simulink library "rappid_564xl_ec_toolbox"  (R2016b)
settings: Solver=FixedStepDiscrete  StartTime=0.0  StopTime=10.0  RelTol=1e-3  EnableMultiTasking=on
undefined symbols (not defined in the file or in its folder): CTU_unit, mem_AddrLW, mem_AddrUP, rappid_564xl_adc_input_support_rev2, rappid_564xl_can_support_rev2, read_mem_AddrLW, read_mem_AddrUP
(part 3 of 6)

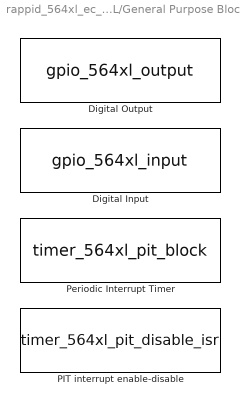
== system rappid_564xl_ec_toolbox/MPC564xL/General Purpose Blocks ==
  Digital Input : S-Function  FunctionName=gpio_564xl_input  Parameters=uint16(pcrNum)  SFunctionDeploymentMode=off  EnableBusSupport=off  mask(GPIO_564xL_Input){gpio_outputs=None, pinNum=None Selected, pcrNum=}
      mask prompts: gpio_outputs "Output Pin (GPI [0-144])"; pinNum "Pin Number"; pcrNum "PCR Number"
      mask help:
      | Select a General Purpose Input Pin as a Source.
      | Output Legend (PCR : Port Name : [ Pin# 144pkg ] : [ Pin# 257pkg ])
      mask init:
      | gpioInfoOut = rappid_564xl_get_gpio_info(gcb);
      | set_param(gcb,'pinNum',gpioInfoOut.pinNum);
      | set_param(gcb,'pcrNum',gpioInfoOut.pcrNum);
      | st=['Pin: ', gpioInfoOut.pinNum,' ',gpioInfoOut.portName,' '];
      mask Help: web([rappid_block_help,filesep,'gpio_input.htm']);
      mask TypeOptions gpio_outputs: 0   : PA0  : [ 73 ] : [ T14 ] | 1   : PA1  : [ 74 ] : [ R14 ] | 2   : PA2  : [ 84 ] : [ N16 ] | 3   : PA3  : [ 92 ] : [ K17 ] | 4   : PA4  : [ 108 ] : [ C16 ] | 5   : PA5  : [ 14 ] : [ H4 ] | 6   : PA6  : [ 2 ] : [ G4 ] | 7   : PA7  : [ 10 ] : [ F3 ] | 8   : PA8  : [ 12 ] : [ F4 ] | 9   : PA9  : [ 134 ] : [ B6 ] | 10  : PA10  : [ 118 ] : [ A13 ] | 11  : PA11 : [ 120 ] : [ D11 ] | 12  : PA12 : [ 122 ] : [ A10 ] | 13  : PA13 : [ 136 ] : [ C6 ] | 14  : PA14 : [ 143 ] : [ B4 ] | 15  : PA15 : [ 144 ] : [ D3 ] | 16  : PB0  : [ 109 ] : [ B15 ] | 17  : PB1  : [ 110 ] : [ C14 ] | 18  : PB2  : [ 114 ] : [ A14 ] | 19  : PB3  : [ 116 ] : [ B13 ] | 20  : PB4  : [ 89 ] : [ L17 ] | 21  : PB5  : [ 86 ] : [ M15 ] | 22  : PB6  : [ 138 ] : [ B3 ] | 23  : PB7  : [ 43 ] : [ R5 ] | 24  : PB8  : [ 47 ] : [ P7 ] | 25  : PB9  : [ 52 ] : [ U7 ] | 26  : PB10 : [ 53 ] : [ R8 ] | 27  : PB11 : [ 54 ] : [ T8 ] | 28  : PB12 : [ 55 ] : [ U8 ] | 29  : PB13 : [ 60 ] : [ R10 ] | 30  : PB14 : [ 64 ] : [ P11 ] | 31  : PB15 : [ 62 ] : [ R11 ] | 32  : PC0  : [ 66 ] : [ R12 ] | 33  : PC1  : [ 41 ] : [ T4 ] | 34  : PC2  : [ 45 ] : [ U5 ] | 36  : PC4  : [ 11 ] : [ H3 ] | 37  : PC5  : [ 13 ] : [ G3 ] | 38  : PC6  : [ 142 ] : [ D4 ] | 39  : PC7  : [ 15 ] : [ K4 ] | 42  : PC10 : [ 111 ] : [ A15 ] | 43  : PC11 : [ 80 ] : [ M14 ] | 44  : PC12 : [ 82 ] : [ N15 ] | 45  : PC13 : [ 101 ] : [ F15 ] | 46  : PC14 : [ 103 ] : [ E15 ] | 47  : PC15 : [ 124 ] : [ A8 ] | 48  : PD0  : [ 125 ] : [ B8 ] | 49  : PD1  : [ 3 ] : [ E3 ] | 50  : PD2  : [ 140 ] : [ C5 ] | 51  : PD3  : [ 128 ] : [ A7 ] | 52  : PD4  : [ 129 ] : [ B7 ] | 53  : PD5  : [ 33 ] : [ N3 ] | 54  : PD6  : [ 34 ] : [ P3 ] | 55  : PD7  : [ 37 ] : [ R4 ] | 56  : PD8  : [ 32 ] : [ M3 ] | 57  : PD9  : [ 26 ] : [ L3 ] | 58  : PD10 : [ 76 ] : [ T15 ] | 59  : PD11 : [ 78 ] : [ R16 ] | 60  : PD12 : [ 99 ] : [ G14 ] | 62  : PD14 : [ 105 ] : [ D16 ] | 64  : PE0  : [ 68 ] : [ T13 ] | 66  : PE2  : [ 49 ] : [ U6 ] | 68  : PE4  : [ 42 ] : [ U4 ] | 69  : PE5  : [ 44 ] : [ T5 ] | 70  : PE6  : [ 46 ] : [ R6 ] | 71  : PE7  : [ 48 ] : [ T6 ] | 73  : PE9  : [ 61 ] : [ T10 ] | 74  : PE10 : [ 63 ] : [ T11 ] | 75  : PE11 : [ 65 ] : [ U11 ] | 76  : PE12 : [ 67 ] : [ T12 ] | 77  : PE13 : [ 117 ] : [ D12 ] | 78  : PE14 : [ 119 ] : [ B12 ] | 79  : PE15 : [ 121 ] : [ B11 ] | 80  : PF0  : [ 133 ] : [ D7 ] | 83  : PF3  : [ 139 ] : [ B5 ] | 84  : PF4  : [ 4 ] : [ D2 ] | 85  : PF5  : [ 5 ] : [ D1 ] | 86  : PF6  : [ 8 ] : [ E2 ] | 87  : PF7  : [ 19 ] : [ J1 ] | 88  : PF8  : [ 20 ] : [ K2 ] | 89  : PF9  : [ 23 ] : [ K1 ] | 90  : PF10 : [ 24 ] : [ L1 ] | 91  : PF11 : [ 25 ] : [ L2 ] | 92  : PF12 : [ 106 ] : [ C17 ] | 93  : PF13 : [ 112 ] : [ B14 ] | 94  : PF14 : [ 115 ] : [ C13 ] | 95  : PF15 : [ 113 ] : [ D13 ] | 98  : PG2  : [ 102 ] : [ E16 ] | 99  : PG3  : [ 104 ] : [ D17 ] | 100 : PG4  : [ 100 ] : [ F17 ] | 101 : PG5  : [ 85 ] : [ N17 ] | 102 : PG6  : [ 98 ] : [ G17 ] | 103 : PG7  : [ 83 ] : [ P17 ] | 104 : PG8  : [ 81 ] : [ P16 ] | 105 : PG9  : [ 79 ] : [ R17 ] | 106 : PG10 : [ 77 ] : [ P15 ] | 107 : PG11 : [ 75 ] : [ U15 ] | 108 : PG12 : [ --- ] : [ F2 ] | 109 : PG13 : [ --- ] : [ H1 ] | 110 : PG14 : [ --- ] : [ A6 ] | 111 : PG15 : [ --- ] : [ J2 ] | 112 : PH0  : [ --- ] : [ A5 ] | 113 : PH1  : [ --- ] : [ F1 ] | 114 : PH2  : [ --- ] : [ A4 ] | 115 : PH3  : [ --- ] : [ G1 ] | 116 : PH4  : [ --- ] : [ L16 ] | 117 : PH5  : [ --- ] : [ M17 ] | 118 : PH6  : [ --- ] : [ H17 ] | 119 : PH7  : [ --- ] : [ K16 ] | 120 : PH8  : [ --- ] : [ K15 ] | 121 : PH9  : [ --- ] : [ G16 ] | 122 : PH10 : [ --- ] : [ A11 ] | 123 : PH11 : [ --- ] : [ C11 ] | 124 : PH12 : [ --- ] : [ B10 ] | 125 : PH13 : [ --- ] : [ G15 ] | 126 : PH14 : [ --- ] : [ A12 ] | 127 : PH15 : [ --- ] : [ J17 ] | 128 : PI0  : [ --- ] : [ C9 ] | 129 : PI1  : [ --- ] : [ C12 ] | 130 : PI2  : [ --- ] : [ F16 ] | 131 : PI3  : [ --- ] : [ E17 ] | 132 : PI4  : [ --- ] : [ K3 ] | None
      mask Display:
      | disp(st);
      | port_label('output',1,'input')
  "Digital Output " : S-Function  FunctionName=gpio_564xl_output  Parameters=uint16(pcrNum)  SFunctionDeploymentMode=off  EnableBusSupport=off  mask(GPIO_564xL_Output){gpio_outputs=None, pinNum=None Selected, pcrNum=}
      mask prompts: gpio_outputs "Output Pin (GPO [0-144])"; pinNum "Pin Number"; pcrNum "PCR Number"
      mask help:
      | Select a General Purpose Output Pin as a Sink.
      | Output Legend (PCR : Port Name : [ Pin# 144pkg ] : [ Pin# 257pkg ])
      mask init:
      | gpioInfoOut = rappid_564xl_get_gpio_info(gcb);
      | set_param(gcb,'pinNum',gpioInfoOut.pinNum);
      | set_param(gcb,'pcrNum',gpioInfoOut.pcrNum);
      | st=['Pin: ', gpioInfoOut.pinNum,' ',gpioInfoOut.portName,' '];
      mask Help: web([rappid_block_help,filesep,'gpio_output.htm']);
      mask TypeOptions gpio_outputs: 0   : PA0  : [ 73 ] : [ T14 ] | 1   : PA1  : [ 74 ] : [ R14 ] | 2   : PA2  : [ 84 ] : [ N16 ] | 3   : PA3  : [ 92 ] : [ K17 ] | 4   : PA4  : [ 108 ] : [ C16 ] | 5   : PA5  : [ 14 ] : [ H4 ] | 6   : PA6  : [ 2 ] : [ G4 ] | 7   : PA7  : [ 10 ] : [ F3 ] | 8   : PA8  : [ 12 ] : [ F4 ] | 9   : PA9  : [ 134 ] : [ B6 ] | 10  : PA10  : [ 118 ] : [ A13 ] | 11  : PA11 : [ 120 ] : [ D11 ] | 12  : PA12 : [ 122 ] : [ A10 ] | 13  : PA13 : [ 136 ] : [ C6 ] | 14  : PA14 : [ 143 ] : [ B4 ] | 15  : PA15 : [ 144 ] : [ D3 ] | 16  : PB0  : [ 109 ] : [ B15 ] | 17  : PB1  : [ 110 ] : [ C14 ] | 18  : PB2  : [ 114 ] : [ A14 ] | 19  : PB3  : [ 116 ] : [ B13 ] | 20  : PB4  : [ 89 ] : [ L17 ] | 21  : PB5  : [ 86 ] : [ M15 ] | 22  : PB6  : [ 138 ] : [ B3 ] | 23  : PB7  : [ 43 ] : [ R5 ] | 24  : PB8  : [ 47 ] : [ P7 ] | 25  : PB9  : [ 52 ] : [ U7 ] | 26  : PB10 : [ 53 ] : [ R8 ] | 27  : PB11 : [ 54 ] : [ T8 ] | 28  : PB12 : [ 55 ] : [ U8 ] | 29  : PB13 : [ 60 ] : [ R10 ] | 30  : PB14 : [ 64 ] : [ P11 ] | 31  : PB15 : [ 62 ] : [ R11 ] | 32  : PC0  : [ 66 ] : [ R12 ] | 33  : PC1  : [ 41 ] : [ T4 ] | 34  : PC2  : [ 45 ] : [ U5 ] | 36  : PC4  : [ 11 ] : [ H3 ] | 37  : PC5  : [ 13 ] : [ G3 ] | 38  : PC6  : [ 142 ] : [ D4 ] | 39  : PC7  : [ 15 ] : [ K4 ] | 42  : PC10 : [ 111 ] : [ A15 ] | 43  : PC11 : [ 80 ] : [ M14 ] | 44  : PC12 : [ 82 ] : [ N15 ] | 45  : PC13 : [ 101 ] : [ F15 ] | 46  : PC14 : [ 103 ] : [ E15 ] | 47  : PC15 : [ 124 ] : [ A8 ] | 48  : PD0  : [ 125 ] : [ B8 ] | 49  : PD1  : [ 3 ] : [ E3 ] | 50  : PD2  : [ 140 ] : [ C5 ] | 51  : PD3  : [ 128 ] : [ A7 ] | 52  : PD4  : [ 129 ] : [ B7 ] | 53  : PD5  : [ 33 ] : [ N3 ] | 54  : PD6  : [ 34 ] : [ P3 ] | 55  : PD7  : [ 37 ] : [ R4 ] | 56  : PD8  : [ 32 ] : [ M3 ] | 57  : PD9  : [ 26 ] : [ L3 ] | 58  : PD10 : [ 76 ] : [ T15 ] | 59  : PD11 : [ 78 ] : [ R16 ] | 60  : PD12 : [ 99 ] : [ G14 ] | 62  : PD14 : [ 105 ] : [ D16 ] | 64  : PE0  : [ 68 ] : [ T13 ] | 66  : PE2  : [ 49 ] : [ U6 ] | 68  : PE4  : [ 42 ] : [ U4 ] | 69  : PE5  : [ 44 ] : [ T5 ] | 70  : PE6  : [ 46 ] : [ R6 ] | 71  : PE7  : [ 48 ] : [ T6 ] | 73  : PE9  : [ 61 ] : [ T10 ] | 74  : PE10 : [ 63 ] : [ T11 ] | 75  : PE11 : [ 65 ] : [ U11 ] | 76  : PE12 : [ 67 ] : [ T12 ] | 77  : PE13 : [ 117 ] : [ D12 ] | 78  : PE14 : [ 119 ] : [ B12 ] | 79  : PE15 : [ 121 ] : [ B11 ] | 80  : PF0  : [ 133 ] : [ D7 ] | 83  : PF3  : [ 139 ] : [ B5 ] | 84  : PF4  : [ 4 ] : [ D2 ] | 85  : PF5  : [ 5 ] : [ D1 ] | 86  : PF6  : [ 8 ] : [ E2 ] | 87  : PF7  : [ 19 ] : [ J1 ] | 88  : PF8  : [ 20 ] : [ K2 ] | 89  : PF9  : [ 23 ] : [ K1 ] | 90  : PF10 : [ 24 ] : [ L1 ] | 91  : PF11 : [ 25 ] : [ L2 ] | 92  : PF12 : [ 106 ] : [ C17 ] | 93  : PF13 : [ 112 ] : [ B14 ] | 94  : PF14 : [ 115 ] : [ C13 ] | 95  : PF15 : [ 113 ] : [ D13 ] | 98  : PG2  : [ 102 ] : [ E16 ] | 99  : PG3  : [ 104 ] : [ D17 ] | 100 : PG4  : [ 100 ] : [ F17 ] | 101 : PG5  : [ 85 ] : [ N17 ] | 102 : PG6  : [ 98 ] : [ G17 ] | 103 : PG7  : [ 83 ] : [ P17 ] | 104 : PG8  : [ 81 ] : [ P16 ] | 105 : PG9  : [ 79 ] : [ R17 ] | 106 : PG10 : [ 77 ] : [ P15 ] | 107 : PG11 : [ 75 ] : [ U15 ] | 108 : PG12 : [ --- ] : [ F2 ] | 109 : PG13 : [ --- ] : [ H1 ] | 110 : PG14 : [ --- ] : [ A6 ] | 111 : PG15 : [ --- ] : [ J2 ] | 112 : PH0  : [ --- ] : [ A5 ] | 113 : PH1  : [ --- ] : [ F1 ] | 114 : PH2  : [ --- ] : [ A4 ] | 115 : PH3  : [ --- ] : [ G1 ] | 116 : PH4  : [ --- ] : [ L16 ] | 117 : PH5  : [ --- ] : [ M17 ] | 118 : PH6  : [ --- ] : [ H17 ] | 119 : PH7  : [ --- ] : [ K16 ] | 120 : PH8  : [ --- ] : [ K15 ] | 121 : PH9  : [ --- ] : [ G16 ] | 122 : PH10 : [ --- ] : [ A11 ] | 123 : PH11 : [ --- ] : [ C11 ] | 124 : PH12 : [ --- ] : [ B10 ] | 125 : PH13 : [ --- ] : [ G15 ] | 126 : PH14 : [ --- ] : [ A12 ] | 127 : PH15 : [ --- ] : [ J17 ] | 128 : PI0  : [ --- ] : [ C9 ] | 129 : PI1  : [ --- ] : [ C12 ] | 130 : PI2  : [ --- ] : [ F16 ] | 131 : PI3  : [ --- ] : [ E17 ] | 132 : PI4  : [ --- ] : [ K3 ] | None
      mask Display:
      | disp(st);
      | port_label('input',1,'output')
  PIT interrupt enable-disable : S-Function  FunctionName=timer_564xl_pit_disable_isr  Parameters=char(pit_chan), uint16(pit_interr)  SFunctionDeploymentMode=off  EnableBusSupport=off  mask(PIT_564xL_isr_enable){pit_chan=1, pit_interr=off}
      mask prompts: pit_chan "PIT Channel (1-3)"; pit_interr "Enable Timer Interrupt"
      mask help: This block enables or disables the interrupt for each PIT block.
      mask init:
      | crlf = sprintf('\n');
      | pit_ch = get_param(gcb, 'pit_chan');
      | 
      | int_stat = get_param(gcb, 'pit_interr');
      | 
      | maskStr = [ 'Periodic Interrupt Timer', crlf, 'Channel ',pit_ch, crlf,'PIT interrupt: ', int_stat];
      mask Help: web([rappid_block_help,filesep,'timer_pit_isr_en.htm']);
      mask TypeOptions pit_chan: 1 | 2 | 3
      mask Display: disp(maskStr)
  Periodic Interrupt Timer : S-Function  InitFcn=|  FunctionName=timer_564xl_pit_block  Parameters=char(pit_chan),uint32(pit_timeout_val)  SFunctionDeploymentMode=off  EnableBusSupport=off  mask(timer_564xl_pit_block){pit_chan=1, pit_timeout=100, int_priority=12, pit_timeout_val=11999999}
      | [pitChan,pitTimeout,timeOutVal]=rappid_564xl_pit_block_update(gcb);
      | rappid_564xl_set_isr_cg_block_att(gcb);
      mask prompts: pit_chan "PIT Channel (1-3)"; pit_timeout "PIT Timeout Value (ms)"; int_priority "Interrupt Priority (0-15)"; pit_timeout_val "Time Out Stored Integer Value"
      mask help: This block triggers an interrupt routine to execute every timeout of this periodic interrupt timer channel.
      mask init:
      | crlf = sprintf('\n');
      | [pitChan,pitTimeout,timeOutVal]=rappid_564xl_pit_block_update(gcb);
      | intPri = get_param(gcb,'int_priority');
      | maskStr = [ 'Periodic Interrupt Timer',crlf, 'Channel ',pitChan, crlf, pitTimeout, ' ms',crlf,'Interrupt Priority ',intPri];
      mask Help: web([rappid_block_help,filesep,'timer_pit.htm']);
      mask TypeOptions pit_chan: 1 | 2 | 3
      mask TypeOptions int_priority: 0 | 1 | 2 | 3 | 4 | 5 | 6 | 7 | 8 | 9 | 10 | 11 | 12 | 13 | 14 | 15
      mask Display:
      | disp(maskStr)
      | port_label('output',1,'trigger')
